simulink model "Differential_steer_kinematic"  (R2019a)
settings: Solver=FixedStepAuto  StartTime=0.0  StopTime=100  FixedStep=.001  RelTol=1e-3
values from neighbouring files (symbols this model uses):
  init = [0,0,0]    [Jackal_kinematic_model.m]
  speed = 1.5    [JACKAL_dynamic_model.m]    (also in Jackal_kinematic_model.m = 2)
  width = basesize(2)    [JACKAL_dynamic_model.m]    (also in Jackal_kinematic_model.m = 0.323)
libraries: fuzblock x1, simulink x1
settings Model: Creator=12248  LastModifiedBy=12248

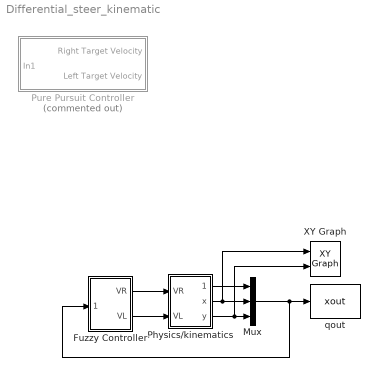
== system Differential_steer_kinematic ==
  Fuzzy Controller : Subsystem
  Mux : Mux  Inputs=3
  Physics/kinematics : Subsystem
  Pure Pursuit Controller : Subsystem  Commented=on
  XY Graph : simulink/Sinks/XY Graph  xmin=-10  xmax=10  ymin=-10  ymax=10  st=-1
  qout : ToWorkspace  VariableName=xout  SampleTime=-1
  wires:
  Mux/1 -> Fuzzy Controller/1(theta,x,y), qout/1
  Physics/kinematics/1(theta) -> Mux/1
  Physics/kinematics/2(x) -> XY Graph/1, Mux/2
  Physics/kinematics/3(y) -> XY Graph/2, Mux/3
  Fuzzy Controller/2(VL) -> Physics/kinematics/2(VL)
  Fuzzy Controller/1(VR) -> Physics/kinematics/1(VR)

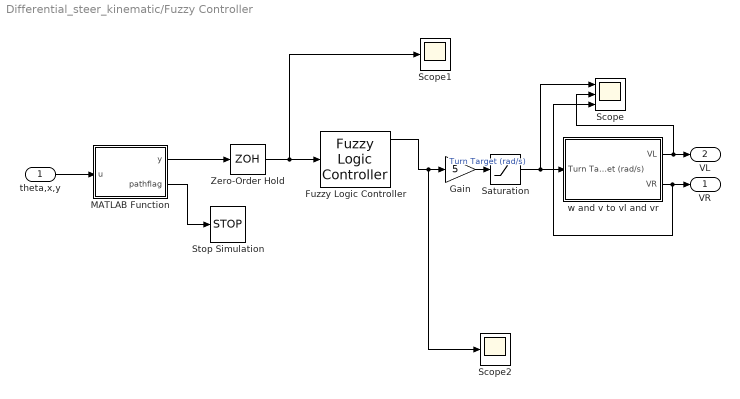
== system Differential_steer_kinematic/Fuzzy Controller ==
  theta,x,y : Inport
  Fuzzy Logic Controller : fuzblock/Fuzzy Logic  Controller  FIS='anfis_kin2.fis'  OutputSampleNumber=3000  DataType=double  FuzzifiedInputs=off  RuleFiringStrengths=on  RuleOutputs=off  AggregatedOutputs=on  SimulateUsing=Code generation  OutOfRangeInputValueMessage=warning  NoRuleFiredMessage=warning  EmptyOutputFuzzySetMessage=warning
  Gain : Gain  Gain=5
  MATLAB Function : MATLAB Function  TreatAsAtomicUnit=on
  Saturation : Saturate  UpperLimit=pi  LowerLimit=-pi
  Scope : Scope  NumInputPorts=3
  Scope1 : Scope
  Scope2 : Scope
  Stop Simulation : Stop
  Zero-Order Hold : ZeroOrderHold  SampleTime=.001
  w and v to vl and vr : Subsystem
  VR : Outport
  VL : Outport  Port=2
  wires:
  Fuzzy Logic Controller/1 -> Scope2/1, Gain/1
  w and v to vl and vr/1(VL) -> Scope/2, VL/1
  w and v to vl and vr/2(VR) -> Scope/3, VR/1
  theta,x,y/1 -> MATLAB Function/1(u)
  MATLAB Function/1(y) -> Zero-Order Hold/1
  MATLAB Function/2(pathflag) -> Stop Simulation/1
  Zero-Order Hold/1 -> Scope1/1, Fuzzy Logic Controller/1
  Saturation/1 -> Scope/1, w and v to vl and vr/1(Turn Target (rad/s))
  Gain/1 -> Saturation/1  "Turn Target (rad/s)"

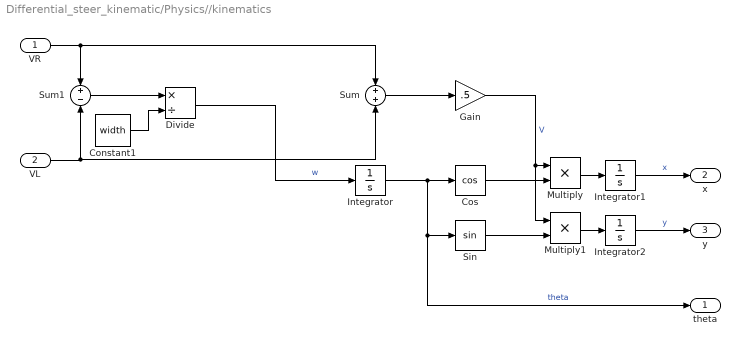
== system Differential_steer_kinematic/Physics//kinematics ==
  VR : Inport
  VL : Inport  Port=2
  Constant1 : Constant  Value=width
  Cos : Trigonometry  Operator=cos
  Divide : Product  Inputs=*/
  Gain : Gain  Gain=.5
  Integrator : Integrator  InitialCondition=init(1)
  Integrator1 : Integrator  InitialCondition=init(2)
  Integrator2 : Integrator  InitialCondition=init(3)
  Multiply : Product
  Multiply1 : Product
  Sin : Trigonometry
  Sum : Sum  Inputs=+|+
  Sum1 : Sum  Inputs=+|-
  theta : Outport
  x : Outport  Port=2
  y : Outport  Port=3
  wires:
  Sin/1 -> Multiply1/2
  Gain/1 -> Multiply1/1, Multiply/1  "V"
  Multiply1/1 -> Integrator2/1
  Integrator/1 -> theta/1, Sin/1, Cos/1  "theta"
  Cos/1 -> Multiply/2
  Multiply/1 -> Integrator1/1
  Divide/1 -> Integrator/1  "w"
  VR/1 -> Sum/1, Sum1/1
  VL/1 -> Sum1/2, Sum/2
  Sum/1 -> Gain/1
  Constant1/1 -> Divide/2
  Sum1/1 -> Divide/1
  Integrator1/1 -> x/1  "x"
  Integrator2/1 -> y/1  "y"

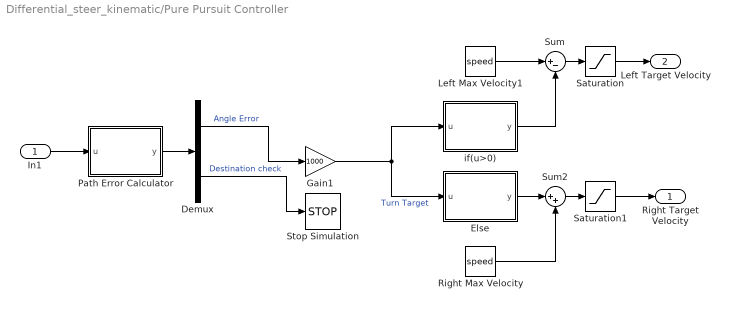
== system Differential_steer_kinematic/Pure Pursuit Controller ==
  In1 : Inport
  Demux : Demux  Outputs=2
  Else : MATLAB Function  TreatAsAtomicUnit=on
  Gain1 : Gain  Gain=1000
  Left Max Velocity1 : Constant  Value=speed
  Path Error Calculator : MATLAB Function  TreatAsAtomicUnit=on
  Right Max Velocity : Constant  Value=speed
  Saturation : Saturate  UpperLimit=speed  LowerLimit=-speed
  Saturation1 : Saturate  UpperLimit=speed  LowerLimit=-speed
  Stop Simulation : Stop
  Sum : Sum  Inputs=|+-
  Sum2 : Sum  Inputs=|++
  if(u>0) : MATLAB Function  TreatAsAtomicUnit=on
  Right Target Velocity : Outport
  Left Target Velocity : Outport  Port=2
  wires:
  Path Error Calculator/1(y) -> Demux/1
  In1/1 -> Path Error Calculator/1(u)
  Gain1/1 -> if(u>0)/1(u), Else/1(u)  "Turn Target"
  Left Max Velocity1/1 -> Sum/1
  Right Max Velocity/1 -> Sum2/2
  if(u>0)/1(y) -> Sum/2
  Sum/1 -> Saturation/1
  Saturation/1 -> Left Target Velocity/1
  Sum2/1 -> Saturation1/1
  Saturation1/1 -> Right Target Velocity/1
  Demux/2 -> Stop Simulation/1  "Destination check"
  Demux/1 -> Gain1/1  "Angle Error"
  Else/1(y) -> Sum2/1

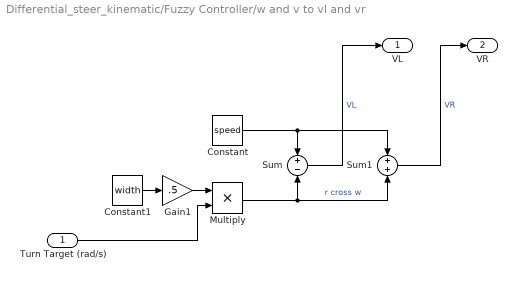
== system Differential_steer_kinematic/Fuzzy Controller/w and v to vl and vr ==
  Turn Target (rad/s) : Inport
  Constant : Constant  Value=speed
  Constant1 : Constant  Value=width
  Gain1 : Gain  Gain=.5
  Multiply : Product  Inputs=**
  Sum : Sum  Inputs=+|-
  Sum1 : Sum  Inputs=+|+
  VL : Outport
  VR : Outport  Port=2
  wires:
  Multiply/1 -> Sum/2, Sum1/2  "r cross w"
  Sum1/1 -> VR/1  "VR"
  Sum/1 -> VL/1  "VL"
  Turn Target (rad/s)/1 -> Multiply/2
  Constant1/1 -> Gain1/1
  Gain1/1 -> Multiply/1
  Constant/1 -> Sum1/1, Sum/1

== matlab function Differential_steer_kinematic/Pure Pursuit Controller/Path Error Calculator ==
  data: u input; y output
%the goal of this script is to check where the robot needs to go (via
%looking at path stepoints) and if the robot needs to travel towards a
%setpoint, it calculates the difference between the robot's actual heading
%and what its desired heading should be to reach that point while traveling
%in a straight line.

function y = fcn(u)
coder.extrinsic('evalin', 'assignin');
pathcount = 0; pathlength=0; % Needed in order to set variable class correctly

pathcount = evalin('base','pathcount'); % Read pathcount from workspace             
pathlength = evalin('base','pathlength'); % Read pathlength from workspace   

path=zeros(pathlength,2);
path = evalin('base','path'); % Read path from workspace

pathflag=0; %flag to stop sim when all points are reached
[len,~]=size(path);
path=[path; 500 500];

pos=[u(2) u(3)]; % [x,y]
currentAngle=u(1); % theta

target=path(pathcount+1,:); %target point is the next point in the path
distErr=sqrt((target(1)-pos(1))^2+(target(2)-pos(2))^2);

if(distErr<.35)
    pathcount=pathcount+1;
    target=path(pathcount+1,:);
    assignin('base','pathcount',pathcount); % Assign new pathcount back to workspace
end

targetAngle=atan2(target(2)-pos(2),target(1)-pos(1)); % Angle between current robot position and the target
angErr=targetAngle-currentAngle;
    
if(angErr>pi()) %keep error between -pi and pi
    angErr=angErr-2*pi();
end

if(angErr<(-1*pi()))
    angErr=angErr+2*pi();
end

if(pathcount>=len) %if all of the target points have been reached
    pathflag=1;
end

y=[angErr pathflag];

== matlab function Differential_steer_kinematic/Fuzzy Controller/MATLAB Function ==
  settings: updateMethod=DISCRETE
  data: u input; y output; pathflag output
function [y,pathflag] = fcn(u)
coder.extrinsic('evalin', 'assignin');
coder.extrinsic('angdiff');

persistent pathcount;
persistent pathlength;
persistent path; %error in code, initially used path but this is already a matlab function

if isempty(pathcount)
    pathcount=1;
end

if isempty(pathlength)
    
    pathlength=0;
    pathlength = evalin('base','pathlength');
    
    path=zeros(pathlength,2);
    path= evalin('base','path'); % Read path from workspace
    path=[path; path(pathlength,1)+100 path(pathlength,2)+100]; %sim takes multiple iterations to stop after reaching final point, so this prevents it from breaking
end

pos=[u(2) u(3)]; % [x,y] 

coder.extrinsic('wrapToPi');
currentAngle=0;
currentAngle= wrapToPi(u(1));

pathflag=0; %flag to stop sim when all points are reached
currentPoint=path(pathcount,:);
target=path(pathcount+1,:);

distErr=sqrt((target(1)-pos(1))^2+(target(2)-pos(2))^2);

A = [(currentPoint(2)-target(2)), target(1)-currentPoint(1); target(1)-currentPoint(1), target(2)-currentPoint(2)];
b = [ target(1)*currentPoint(2)-currentPoint(1)*target(2); pos(1)*(target(1)-currentPoint(1)) + pos(2)*(target(2)-currentPoint(2))];
proj = (A\b)'; %projected point on the line between  .
projLen=dot(proj-currentPoint,target-currentPoint)/norm(target-currentPoint)^2; %the distance along the projected line, where 0 is the start point and 1 is the end point

if ((projLen>1))
    pathcount=pathcount+1;
   
    currentPoint=path(pathcount,:);
    target=path(pathcount+1,:);
end

%check if at destination and terminate sim if there
if (pathcount==pathlength)
    pathflag=1;
end

if ((pathcount==(pathlength-1))||(pathcount==(pathlength)))
    a=path(pathcount,:);
    b=path(pathcount+1,:);
    post=path(pathcount+1,:);
else
    a=path(pathcount,:);
    b=path(pathcount+1,:);
    post=path(pathcount+2,:);
end

th1 = atan2(b(2)-pos(2), b(1)-pos(1));
th2 = atan2(b(2)-a(2), b(1)-a(1));
th3 = atan2(post(2)-b(2), post(1)-b(1)); 

ThetaFA=0;
Theta0=0;
ThetaNext=0;

ThetaFA=angdiff(currentAngle,th1);
Theta0=angdiff(currentAngle,th2);
ThetaNext=angdiff(currentAngle,th3);

d = ( pos(1)-currentPoint(1) )*(target(2)-currentPoint(2)) - (pos(2)-currentPoint(2))*(target(1)-currentPoint(1));

if ( d >0)
    side = 1;
elseif ( d < 0)
    side = -1;
else
    side = 0;
end

distanceError=norm(pos-proj)*side;

%y = [ThetaFA;Theta0;distanceError;ThetaNext];
y = [distanceError;ThetaFA;Theta0];

== matlab function Differential_steer_kinematic/Pure Pursuit Controller/if(u>0) ==
  data: u input; y output
function y = fcn(u)
if(u>0)
    y = u;
else
    y=0;
end

== matlab function Differential_steer_kinematic/Pure Pursuit Controller/Else ==
  data: u input; y output
function y = fcn(u)
if(u<=0)
    y=u;
else
    y=0;
end
